simulink model "Claculator_subsystem"  (R2018a)
settings: Solver=FixedStepDiscrete  StartTime=0.0  StopTime=10.0  RelTol=1e-3
settings Model: Creator=Ahmed Yehia  LastModifiedBy=Ahmed Yehia
settings OptimizationCC: DefaultParameterBehavior=Inlined  EnhancedBackFolding=on  PassReuseOutputArgsAs=Individual arguments  OptimizeBlockOrder=speed  DifferentSizesBufferReuse=on  OptimizationCustomize=off
settings DebuggingCC: UnderspecifiedInitializationDetection=Classic  MergeDetectMultiDrivingBlocksExec=none  ParameterTunabilityLossMsg=error
settings ModelReferenceCC: PropagateSignalLabelsOutOfModel=off
settings SFSimCC: MATLABDynamicMemAlloc=off
settings RTWCC: SystemTargetFile=ert.tlc  GenCodeOnly=on  TemplateMakefile=ert_default_tmf  GenerateReport=on  IncludeHyperlinkInReport=on  LaunchReport=on  GenerateTraceInfo=on  GenerateTraceReport=on  GenerateTraceReportSl=on  GenerateTraceReportSf=on  GenerateTraceReportEml=on
settings CodeAppCC: ForceParamTrailComments=on  IgnoreCustomStorageClasses=off  OperatorAnnotations=on  SimulinkDataObjDesc=on  SFDataObjDesc=on  InsertBlockDesc=on
settings ERTTargetCC: TargetLangStandard=C99 (ISO)  GenerateSampleERTMain=on  InlinedParameterPlacement=NonHierarchical  ERTCustomFileTemplate=example_file_process.tlc

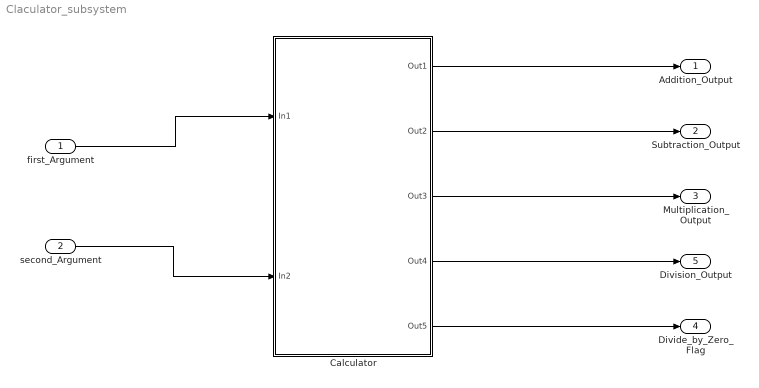
== system Claculator_subsystem ==
  first_Argument : Inport  OutDataTypeStr=double
  second_Argument : Inport  Port=2  OutDataTypeStr=double
  Calculator : Subsystem  TreatAsAtomicUnit=on
      settings: MinAlgLoopOccurrences=on  RTWFcnNameOpts=Use subsystem name
  Addition_Output : Outport  OutDataTypeStr=double
  Subtraction_Output : Outport  Port=2  OutDataTypeStr=double
  Multiplication_Output : Outport  Port=3  OutDataTypeStr=double
  Divide_by_Zero_Flag : Outport  Port=4  OutDataTypeStr=boolean
  Division_Output : Outport  Port=5  OutDataTypeStr=double
  wires:
  first_Argument/1 -> Calculator/1(In1)
  second_Argument/1 -> Calculator/2(In2)
  Calculator/1(Out1) -> Addition_Output/1
  Calculator/2(Out2) -> Subtraction_Output/1
  Calculator/3(Out3) -> Multiplication_Output/1
  Calculator/4(Out4) -> Division_Output/1
  Calculator/5(Out5) -> Divide_by_Zero_Flag/1

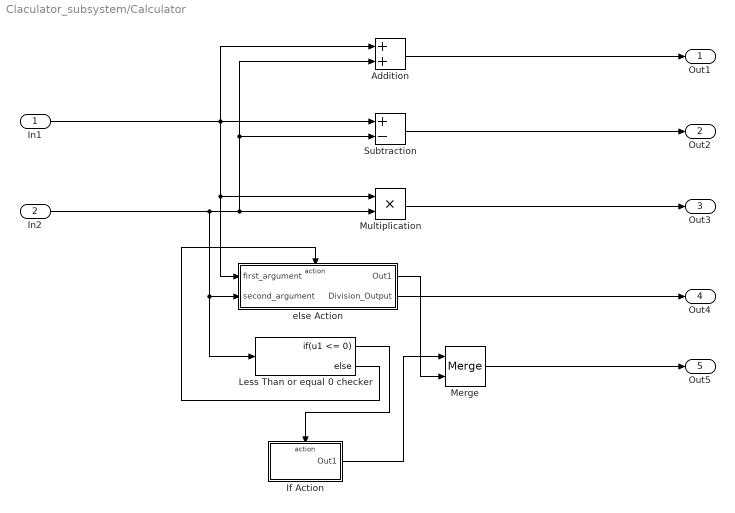
== system Claculator_subsystem/Calculator ==
  In1 : Inport
  In2 : Inport  Port=2
  Addition : Sum  AccumDataTypeStr=double  OutDataTypeStr=double
  If Action : Subsystem  TreatAsAtomicUnit=on
  Less Than or equal 0 checker : If  IfExpression=u1 <= 0
  Merge : Merge
  Multiplication : Product  OutDataTypeStr=double
  Subtraction : Sum  Inputs=+-  AccumDataTypeStr=double  OutDataTypeStr=double
  else Action : Subsystem  TreatAsAtomicUnit=on
  Out1 : Outport
  Out2 : Outport  Port=2
  Out3 : Outport  Port=3
  Out4 : Outport  Port=4
  Out5 : Outport  Port=5
  wires:
  In1/1 -> Subtraction/1, Multiplication/1, else Action/1(first_argument), Addition/1
  else Action/1(Out1) -> Merge/2
  If Action/1(Out1) -> Merge/1
  Subtraction/1 -> Out2/1
  Multiplication/1 -> Out3/1
  In2/1 -> Multiplication/2, Subtraction/2, Addition/2, else Action/2(second_argument), Less Than or equal 0 checker/1
  Less Than or equal 0 checker/2 -> else Action/Action
  Less Than or equal 0 checker/1 -> If Action/Action
  Addition/1 -> Out1/1
  Merge/1 -> Out5/1
  else Action/2(Division_Output) -> Out4/1

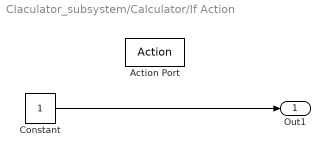
== system Claculator_subsystem/Calculator/If Action ==
  Action Port : ActionPort  ActionType=then
  Constant : Constant  OutDataTypeStr=boolean
  Out1 : Outport  OutDataTypeStr=boolean
  wires:
  Constant/1 -> Out1/1

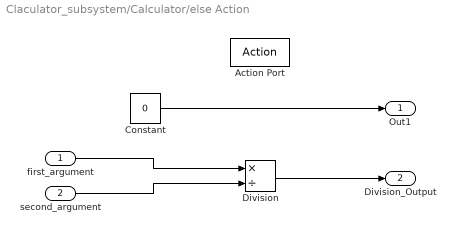
== system Claculator_subsystem/Calculator/else Action ==
  first_argument : Inport  OutDataTypeStr=double
  second_argument : Inport  Port=2  OutDataTypeStr=double
  Action Port : ActionPort  ActionType=else
  Constant : Constant  Value=0  OutDataTypeStr=boolean
  Division : Product  Inputs=*/  OutDataTypeStr=double
  Out1 : Outport  OutDataTypeStr=boolean
  Division_Output : Outport  Port=2  OutDataTypeStr=double
  wires:
  Constant/1 -> Out1/1
  Division/1 -> Division_Output/1
  second_argument/1 -> Division/2
  first_argument/1 -> Division/1
